simulink library "libAeroForceMomentCalcs"  (R2020b)
settings: Solver=VariableStepAuto  StartTime=0.0  StopTime=10.0  RelTol=1e-3
undefined symbols (not defined in the file): data
libraries: aerolibtransform2 x1
settings Model: Creator=caatay  LastModifiedBy=caatay

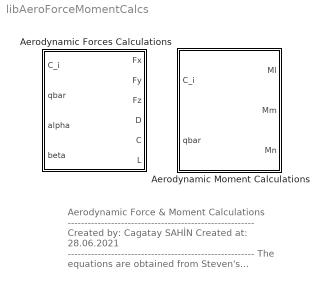
== system libAeroForceMomentCalcs ==
  note: Aerodynamic Force & Moment
      | Calculations
      | --------------------------------------------------------
      | Created by: Cagatay SAHİN
      | Created at: 28.06.2021
      | --------------------------------------------------------
      | The equations are obtained from
      | Steven's textbook.
      | The reference article can be found in
      | "references folder".
      | --------------------------------------------------------
      | for question:
      | cagataysahin44@gmail.com
  Aerodynamic Forces Calculations : Subsystem  mask(Aerodynamic Model - Aerodynamic Forces and Moment Calculation - Aerodynamic Force Calculation){S=data.acSpec.wing.S}
      mask prompts: S "Wing Aera"
      mask help: Aerodynamic Force calculation block calculates body axis aerodynamic forces with using atmosphere and aircraft wing information.
      mask Help:
      | This block can calculate body axis aerodynamic forces with using atmosphere and aircraft wing information.
      | Just calculate body axis forces.
      | -------------------------------------------------------------------------------------------------------------------------------------------------
      | Inputs of this block:
      | 	C_{i}: Aerodynamic total ceofficients.
      | 	qbar: Dynamic Pressure in [lb/ft^2].
      | 	S: Wing Reference Area [ft^2].
      | Outputs of this block:
      | 	F_{i}: Body axis forces in i axis.
      | -------------------------------------------------------------------------------------------------------------------------------------------------
      | Equations that in this block can be found in Steven's textbook. This textbook is in "literature" subfolder.
      | for question: "cagataysahin44@gmail.com".
      mask Display:
      | port_label('input',1,'C_{i}','texmode','on');
      | port_label('input',2,'qbar','texmode','on');
      | port_label('input',3,'\alpha','texmode','on');
      | port_label('input',4,'\beta','texmode','on');
      | 
      | port_label('output',1,'F_{x}','texmode','on');
      | port_label('output',2,'F_{y}','texmode','on');
      | port_label('output',3,'F_{z}','texmode','on');
      | port_label('output',4,'D','texmode','on');
      | port_label('output',5,'C','texmode','on');
      | port_label('output',6,'L','texmode','on');
  Aerodynamic Moment Calculations : Subsystem  mask(Aerodynamic Model - Aerodynamic Forces and Moment Calculation - Aerodynamic Moment Calculation){S=data.acSpec.wing.S, b=data.acSpec.wing.b, cbar=data.acSpec.wing.cbar}
      mask prompts: S "Wing Area"; b "Wing Span"; cbar "Mean Aerodynamic Chord"
      mask help: Aerodynamic moment calculation block calculates body axis aerodynamic forces with using atmosphere and aircraft wing information.
      mask Help:
      | This block can calculate body axis aerodynamic moments with using atmosphere and aircraft wing information.
      | -------------------------------------------------------------------------------------------------------------------------------------------------
      | Inputs of this block:
      | 	C_{i}: Aerodynamic total ceofficients.
      | 	qbar: Dynamic Pressure in [lb/ft^2].
      | 	S: Wing Reference Area [ft^2].
      | 	b: Wing Span [ft].
      | 	cbar: Mean Aerodynamic Chord [ft].
      | Outputs of this block:
      | 	M_{i}: Body axis moments in i axis.
      | -------------------------------------------------------------------------------------------------------------------------------------------------
      | Equations that in this block can be found in Steven's textbook. This textbook is in "literature" subfolder.
      | for question: "cagataysahin44@gmail.com".
      mask Display:
      | port_label('input',1,'C_{i}','texmode','on');
      | port_label('input',2,'qbar','texmode','on');
      | 
      | port_label('output',1,'M_{l}','texmode','on');
      | port_label('output',2,'M_{m}','texmode','on');
      | port_label('output',3,'M_{n}','texmode','on');

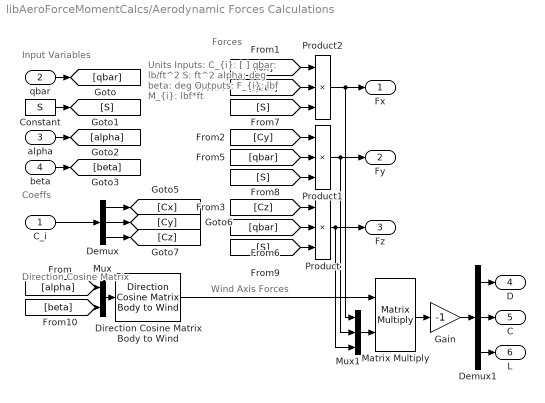
== system libAeroForceMomentCalcs/Aerodynamic Forces Calculations ==
  note: Wind Axis Forces
  note: Direction Cosine Matrix
  note: Coeffs
  note: Forces
  note: Input Variables
  note: Units
      | Inputs:
      | C_{i}: [ ]
      | qbar: lb/ft^2
      | S: ft^2
      | alpha: deg
      | beta: deg
      | Outputs:
      | F_{i}: lbf
      | M_{i}: lbf*ft
  C_i : Inport
  qbar : Inport  Port=2
  alpha : Inport  Port=3
  beta : Inport  Port=4
  Constant : Constant  Value=S
  Demux : Demux  Outputs=3
  Demux1 : Demux  Outputs=3
  Direction Cosine Matrix Body to Wind : aerolibtransform2/Direction Cosine Matrix Body to Wind
      settings: SourceProductBaseCode=AE
  Gain : Gain  Gain=-1
  Matrix Multiply : Product  Multiplication=Matrix(*)
  Mux : Mux  Inputs=2
  Mux1 : Mux  Inputs=3
  Product : Product  Inputs=3
  Product1 : Product  Inputs=3
  Product2 : Product  Inputs=3
  Fx : Outport  VectorParamsAs1DForOutWhenUnconnected=off
  Fy : Outport  Port=2  VectorParamsAs1DForOutWhenUnconnected=off
  Fz : Outport  Port=3  VectorParamsAs1DForOutWhenUnconnected=off
  D : Outport  Port=4  VectorParamsAs1DForOutWhenUnconnected=off
  C : Outport  Port=5  VectorParamsAs1DForOutWhenUnconnected=off
  L : Outport  Port=6  VectorParamsAs1DForOutWhenUnconnected=off
  wires:
  qbar/1 -> [qbar]
  Constant/1 -> [S]
  Demux/1 -> [Cx]
  Demux/2 -> [Cy]
  Demux/3 -> [Cz]
  [S] -> Product/3
  [qbar] -> Product/2
  [Cz] -> Product/1
  [S] -> Product2/3
  [qbar] -> Product2/2
  [Cx] -> Product2/1
  [Cy] -> Product1/1
  [qbar] -> Product1/2
  [S] -> Product1/3
  Product2/1 -> Fx/1, Mux1/1
  Product1/1 -> Fy/1, Mux1/2
  Product/1 -> Fz/1, Mux1/3
  C_i/1 -> Demux/1
  alpha/1 -> [alpha]
  beta/1 -> [beta]
  [alpha] -> Mux/1
  [beta] -> Mux/2
  Mux/1 -> Direction Cosine Matrix Body to Wind/1
  Direction Cosine Matrix Body to Wind/1 -> Matrix Multiply/1
  Mux1/1 -> Matrix Multiply/2
  Matrix Multiply/1 -> Gain/1
  Gain/1 -> Demux1/1
  Demux1/1 -> D/1
  Demux1/2 -> C/1
  Demux1/3 -> L/1

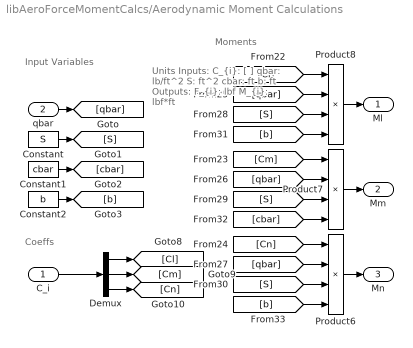
== system libAeroForceMomentCalcs/Aerodynamic Moment Calculations ==
  note: Moments
  note: Input Variables
  note: Coeffs
  note: Units
      | Inputs:
      | C_{i}: [ ]
      | qbar: lb/ft^2
      | S: ft^2
      | cbar: ft
      | b: ft
      | Outputs:
      | F_{i}: lbf
      | M_{i}: lbf*ft
  C_i : Inport
  qbar : Inport  Port=2
  Constant : Constant  Value=S
  Constant1 : Constant  Value=cbar
  Constant2 : Constant  Value=b
  Demux : Demux  Outputs=3
  Product6 : Product  Inputs=4
  Product7 : Product  Inputs=4
  Product8 : Product  Inputs=4
  Ml : Outport  VectorParamsAs1DForOutWhenUnconnected=off
  Mm : Outport  Port=2  VectorParamsAs1DForOutWhenUnconnected=off
  Mn : Outport  Port=3  VectorParamsAs1DForOutWhenUnconnected=off
  wires:
  [qbar] -> Product7/2
  Constant1/1 -> [cbar]
  [S] -> Product7/3
  [b] -> Product8/4
  [Cm] -> Product7/1
  [Cn] -> Product6/1
  [S] -> Product6/3
  [cbar] -> Product7/4
  Constant2/1 -> [b]
  Constant/1 -> [S]
  [b] -> Product6/4
  [Cl] -> Product8/1
  [qbar] -> Product6/2
  [qbar] -> Product8/2
  Product8/1 -> Ml/1
  Product7/1 -> Mm/1
  qbar/1 -> [qbar]
  [S] -> Product8/3
  Product6/1 -> Mn/1
  C_i/1 -> Demux/1
  Demux/3 -> [Cn]
  Demux/2 -> [Cm]
  Demux/1 -> [Cl]
